simulink model "Observer"  (R2022b)
settings: Solver=FixedStepAuto  StartTime=0.0  StopTime=10.0  RelTol=1e-3  SampleTimeConstraint=STIndependent
undefined symbols (not defined in the file): NumberSt, NumModules, NumSeries, OCV_Matrix, R0_Matrix, SOC_Vec1, SOC_Vec2, SOH_Vec, Temperature_Vec
settings Model: DataDictionary=Estimators_Dictionary.sldd  Creator=japerez  LastModifiedBy=jgavidia
settings DataIOCC: SaveOutput=off  SaveTime=off
settings DebuggingCC: ParameterPrecisionLossMsg=none

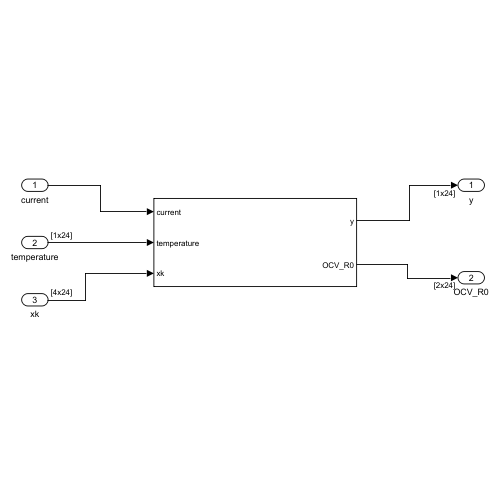
[thumbnail: Simulink's stored preview of the top-level diagram]
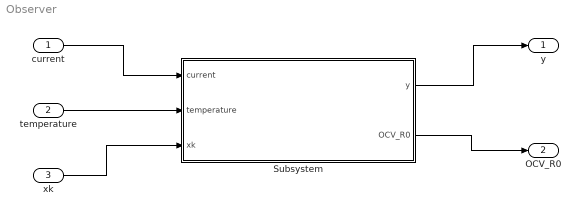
== system Observer ==
  current : Inport  OutDataTypeStr=single  PortDimensions=1
  temperature : Inport  Port=2  OutDataTypeStr=single  PortDimensions=[1,NumModules*NumSeries]
  xk : Inport  Port=3  OutDataTypeStr=single  PortDimensions=[NumberSt,NumModules*NumSeries]
  Subsystem : Subsystem
  y : Outport  OutDataTypeStr=single  PortDimensions=[1,NumModules*NumSeries]
  OCV_R0 : Outport  Port=2  OutDataTypeStr=single  PortDimensions=[2,NumModules*NumSeries]
  wires:
  current/1 -> Subsystem/1(current)
  Subsystem/1(y) -> y/1
  xk/1 -> Subsystem/3(xk)
  temperature/1 -> Subsystem/2(temperature)
  Subsystem/2(OCV_R0) -> OCV_R0/1

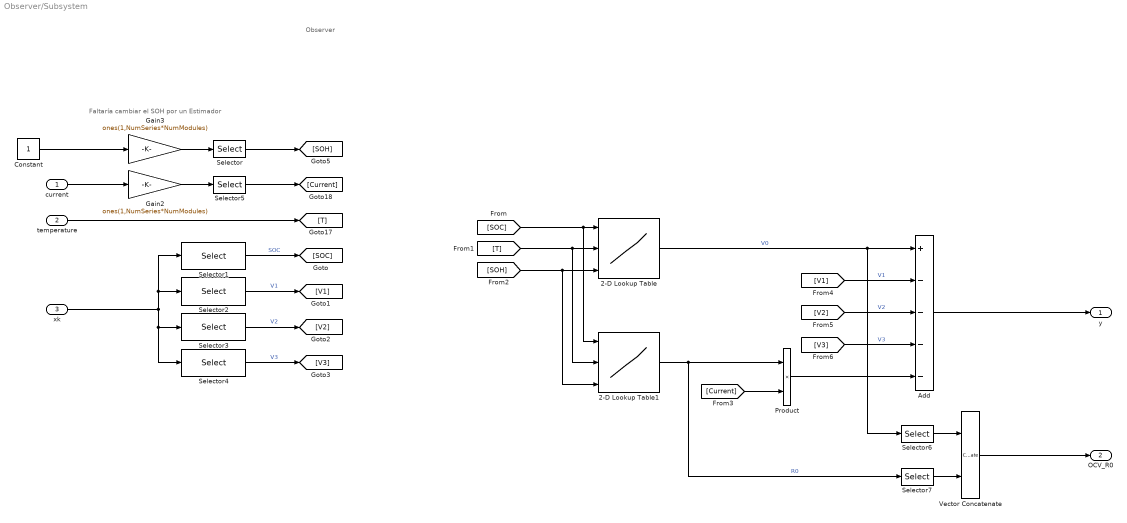
== system Observer/Subsystem ==
  note: Observer
  note: Faltaría cambiar el SOH por un Estimador
  current : Inport
  temperature : Inport  Port=2
  xk : Inport  Port=3
  2-D Lookup Table : Lookup_n-D  NumberOfTableDimensions=3  BreakpointsForDimension1=SOC_Vec1  BreakpointsForDimension2=Temperature_Vec  BreakpointsForDimension3=SOH_Vec  Table=OCV_Matrix  ExtrapMethod=Clip  InternalRulePriority=Speed  RndMeth=Simplest
      settings: InputPortMap=u0,u1,u2
  2-D Lookup Table1 : Lookup_n-D  NumberOfTableDimensions=3  BreakpointsForDimension1=SOC_Vec2  BreakpointsForDimension2=Temperature_Vec  BreakpointsForDimension3=SOH_Vec  Table=R0_Matrix  ExtrapMethod=Clip  InternalRulePriority=Speed  RndMeth=Simplest
      settings: InputPortMap=u0,u1,u2
  Add : Sum  Inputs=+----
  Constant : Constant  OutDataTypeStr=single
  Gain2 : Gain  Gain=ones(1,NumSeries*NumModules)
  Gain3 : Gain  Gain=ones(1,NumSeries*NumModules)
  Product : Product
  Selector{,5..7} (4 alike) : Selector  NumberOfDimensions=2  InputPortWidth=3  IndexOptions=Select all,Index vector (dialog)  Indices=[1 3],[1:24]  OutputSizes=1,1
  Selector1 : Selector  NumberOfDimensions=2  InputPortWidth=24  IndexOptions=Index vector (dialog),Select all  Indices=1,1  OutputSizes=1,1
  Selector2 : Selector  NumberOfDimensions=2  InputPortWidth=24  IndexOptions=Index vector (dialog),Select all  Indices=2,2  OutputSizes=1,1
  Selector3 : Selector  NumberOfDimensions=2  InputPortWidth=24  IndexOptions=Index vector (dialog),Select all  Indices=3,3  OutputSizes=1,1
  Selector4 : Selector  NumberOfDimensions=2  InputPortWidth=24  IndexOptions=Index vector (dialog),Select all  Indices=4,4  OutputSizes=1,1
  Vector Concatenate : Concatenate  Mode=Multidimensional array
  y : Outport
  OCV_R0 : Outport  Port=2
  wires:
  current/1 -> Gain2/1
  Add/1 -> y/1
  temperature/1 -> [T]
  Vector Concatenate/1 -> OCV_R0/1
  Gain2/1 -> Selector5/1
  [V2] -> Add/3  "V2"
  xk/1 -> Selector4/1, Selector3/1, Selector1/1, Selector2/1
  [V1] -> Add/2  "V1"
  [T] -> 2-D Lookup Table/2, 2-D Lookup Table1/2
  [SOC] -> 2-D Lookup Table/1, 2-D Lookup Table1/1
  [Current] -> Product/2
  Selector3/1 -> [V2]  "V2"
  2-D Lookup Table1/1 -> Product/1, Selector7/1  "R0"
  [V3] -> Add/4  "V3"
  Selector2/1 -> [V1]  "V1"
  Gain3/1 -> Selector/1
  Constant/1 -> Gain3/1
  Selector4/1 -> [V3]  "V3"
  [SOH] -> 2-D Lookup Table/3, 2-D Lookup Table1/3
  Selector1/1 -> [SOC]  "SOC"
  Product/1 -> Add/5
  2-D Lookup Table/1 -> Add/1, Selector6/1  "V0"
  Selector/1 -> [SOH]
  Selector5/1 -> [Current]
  Selector6/1 -> Vector Concatenate/1
  Selector7/1 -> Vector Concatenate/2
